simulink model "calcul_alpha_beta_gamma"  (R2024b)
settings: Solver=FixedStepAuto  StartTime=0.0  StopTime=10.0  FixedStep=Ts  RelTol=1e-3
settings Model: Creator=marti  LastModifiedBy=marti

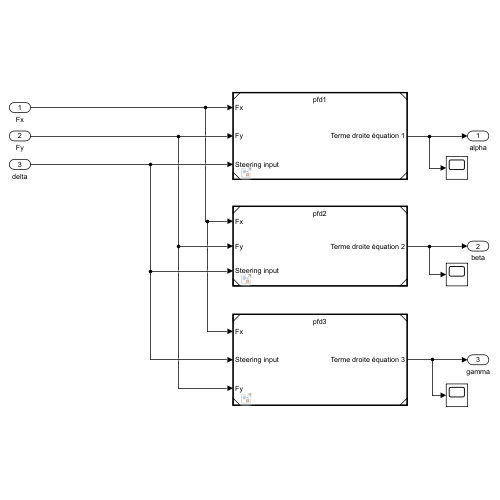
[thumbnail: Simulink's stored preview of the top-level diagram]
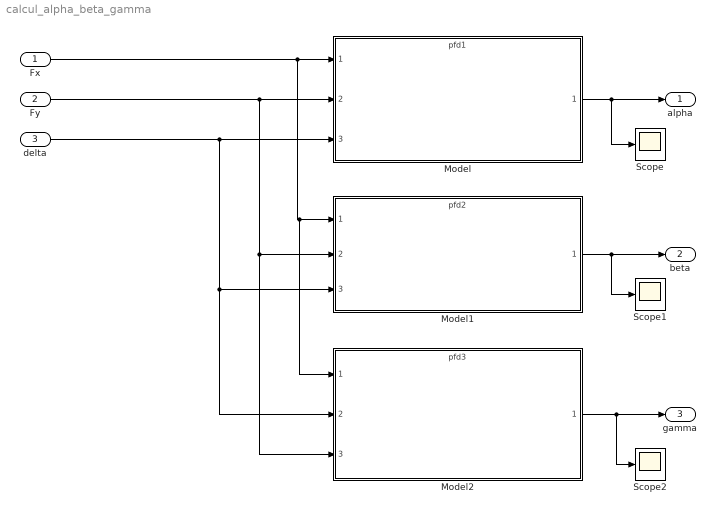
== system calcul_alpha_beta_gamma ==
  Fx : Inport
  Fy : Inport  Port=2
  delta : Inport  Port=3
  Model : ModelReference  ModelNameDialog=pfd1.slx  SimulationMode=Normal  ModelReferenceVersion=1.3
  Model1 : ModelReference  ModelNameDialog=pfd2.slx  SimulationMode=Normal  ModelReferenceVersion=1.3
  Model2 : ModelReference  ModelNameDialog=pfd3.slx  SimulationMode=Normal  ModelReferenceVersion=1.3
  Scope : Scope
  Scope1 : Scope
  Scope2 : Scope
  alpha : Outport
  beta : Outport  Port=2
  gamma : Outport  Port=3
  wires:
  Fx/1 -> Model2/1, Model1/1, Model/1
  Fy/1 -> Model2/3, Model1/2, Model/2
  delta/1 -> Model2/2, Model1/3, Model/3
  Model/1 -> alpha/1, Scope/1
  Model1/1 -> beta/1, Scope1/1
  Model2/1 -> Scope2/1, gamma/1
